simulink model "MBKwithLQDG"  (R2018a)
settings: Solver=ode4  StartTime=0.0  StopTime=50  FixedStep=0.01  RelTol=1e-3
values from neighbouring files (symbols this model uses):
  b = 2    [MBK.m]
  k = 5    [MBK.m]
  m = 10    [MBK.m]
settings Model: Creator=Ali  LastModifiedBy=Ali

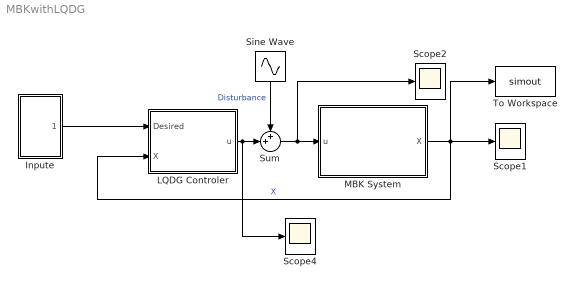
== system MBKwithLQDG ==
  Inpute : Subsystem
  LQDG Controler : Subsystem
  MBK System : Subsystem
  Scope1 : Scope
  Scope2 : Scope
  Scope4 : Scope
  Sine Wave : Sin  SampleTime=0
  Sum : Sum  Inputs=++|
  To Workspace : ToWorkspace  VariableName=simout  SaveFormat=Timeseries  SampleTime=-1
  wires:
  MBK System/1(X) -> To Workspace/1, LQDG Controler/2(X), Scope1/1  "X"
  LQDG Controler/1(u) -> Scope4/1, Sum/2
  Sine Wave/1 -> Sum/1  "Disturbance"
  Sum/1 -> Scope2/1, MBK System/1(u)
  Inpute/1(Desired) -> LQDG Controler/1(Desired)

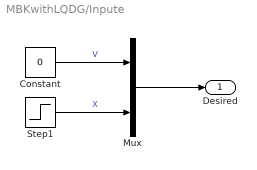
== system MBKwithLQDG/Inpute ==
  Constant : Constant  Value=0
  Mux : Mux  Inputs=2
  Step1 : Step  After=0  SampleTime=0
  Desired : Outport
  wires:
  Mux/1 -> Desired/1
  Step1/1 -> Mux/2  "X"
  Constant/1 -> Mux/1  "V"

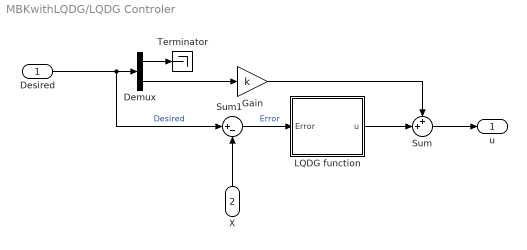
== system MBKwithLQDG/LQDG Controler ==
  Desired : Inport
  X : Inport  Port=2
  Demux : Demux  Outputs=2
  Gain : Gain  Gain=k
  LQDG function : MATLAB Function  TreatAsAtomicUnit=on
  Sum : Sum  Inputs=++|
  Sum1 : Sum  Inputs=|+-
  Terminator : Terminator
  u : Outport
  wires:
  X/1 -> Sum1/2
  LQDG function/1(u) -> Sum/2
  Sum/1 -> u/1
  Sum1/1 -> LQDG function/1(Error)  "Error"
  Gain/1 -> Sum/1
  Desired/1 -> Sum1/1, Demux/1  "Desired"
  Demux/2 -> Gain/1
  Demux/1 -> Terminator/1

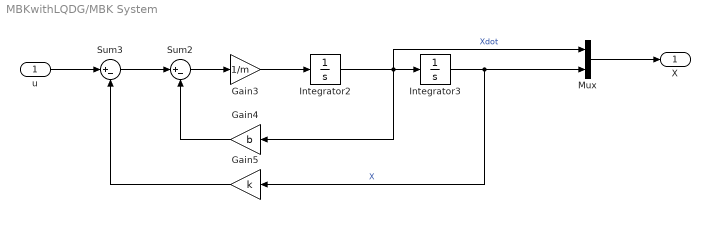
== system MBKwithLQDG/MBK System ==
  u : Inport
  Gain3 : Gain  Gain=1/m
  Gain4 : Gain  Gain=b
  Gain5 : Gain  Gain=k
  Integrator2 : Integrator
  Integrator3 : Integrator  InitialCondition=3
  Mux : Mux  Inputs=2
  Sum2 : Sum  Inputs=|+-
  Sum3 : Sum  Inputs=|+-
  X : Outport
  wires:
  u/1 -> Sum3/1
  Gain4/1 -> Sum2/2
  Gain3/1 -> Integrator2/1
  Integrator3/1 -> Mux/2, Gain5/1  "X"
  Gain5/1 -> Sum3/2
  Sum2/1 -> Gain3/1
  Integrator2/1 -> Mux/1, Gain4/1, Integrator3/1  "Xdot"
  Sum3/1 -> Sum2/1
  Mux/1 -> X/1

== matlab function MBKwithLQDG/LQDG Controler/LQDG function ==
  settings: updateMethod=DISCRETE
  data: u output; Error input
function u = LQDG(Error)
%% System Description
% Mass
m = 10;
% Viscous Friction Coefficient 
b = 2;
% Spring Constant
k = 5;
%% State Space
% x_dot = Ax + Bu - Dv (DV: Disturbance)
%{
A = [ 0    1;
    -k/m -b/m];
C = [0 1];
D = B;
%}
B = [ 0 ;
     1/m];
% Weight Matrix
R = 1;
Q = [5 0;
     0   1] ;
Gamma = 0.8;
%% Riccati Equation
%P * A + A' * P - P * B * R^-1 * B' * P + P * D * Gamma^-1 * D' * P + Q = 0
%P12 Solver
%Q11 - P12 + P12^2/(100*Gamma) - P12^2/(100*R) == 0
a1 = (1 / Gamma - 1 / R) / 100;
b1 = -1;
c1 = Q(1, 1);
Delta1 = b1^2 - 4 * a1 * c1;
P12 = min((-b1 - sqrt(Delta1)) / (2*a1), (-b1 + sqrt(Delta1)) / (2*a1));
%P22 Solver
%2*P12 - (2*P22)/5 + Q22 + P22^2/(100*Gamma) - P22^2/(100*R) == 0
a2 = (1 / Gamma - 1 / R) / 100;
b2 = -2 / 5;
c2 = Q(2, 2) + 2 * P12;
Delta2 = b2^2 - 4 * a2 * c2;
P22 = min((-b2 - sqrt(Delta2)) / (2*a2), (-b2 + sqrt(Delta2)) / (2*a2));
%%P11 Solver
% P11 - P12/5 - P22/2 + (P12*P22)/(100*Gamma) - (P12*P22)/(100*R) == 0
P11 = P12 / 5 + P22 / 2 - P12 * P22 * (1 / Gamma - 1 / R) / 100;
P = [P11 P12;
     P12 P22];
u = -(R^-1)*B'*P*Error;
